simulink model "Control logic"  (R2022a)
settings: Solver=VariableStepAuto  StartTime=0.0  StopTime=10.0  RelTol=1e-3
settings Model: Creator=jbn04  LastModifiedBy=jbn04

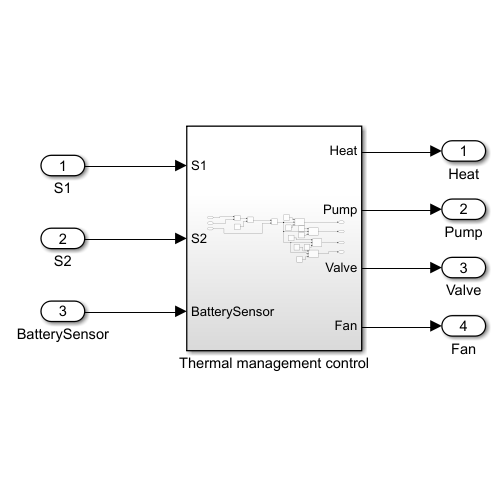
[thumbnail: Simulink's stored preview of the top-level diagram]
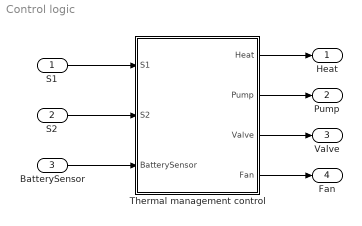
== system Control logic ==
  S1 : Inport
  S2 : Inport  Port=2
  BatterySensor : Inport  Port=3
  Thermal management control : Subsystem
  Heat : Outport
  Pump : Outport  Port=2
  Valve : Outport  Port=3
  Fan : Outport  Port=4
  wires:
  S1/1 -> Thermal management control/1(S1)
  S2/1 -> Thermal management control/2(S2)
  BatterySensor/1 -> Thermal management control/3(BatterySensor)
  Thermal management control/1(Heat) -> Heat/1
  Thermal management control/2(Pump) -> Pump/1
  Thermal management control/3(Valve) -> Valve/1
  Thermal management control/4(Fan) -> Fan/1

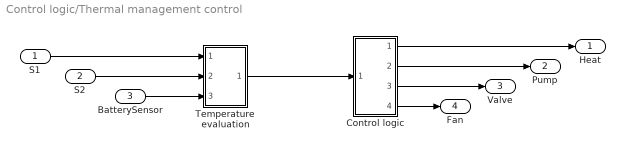
== system Control logic/Thermal management control ==
  S1 : Inport
  S2 : Inport  Port=2
  BatterySensor : Inport  Port=3
  Control logic : Subsystem
  Temperature evaluation : Subsystem
  Heat : Outport
  Pump : Outport  Port=2
  Valve : Outport  Port=3
  Fan : Outport  Port=4
  wires:
  S1/1 -> Temperature evaluation/1(In1)
  S2/1 -> Temperature evaluation/2(In2)
  BatterySensor/1 -> Temperature evaluation/3(In3)
  Temperature evaluation/1(Out1) -> Control logic/1(In1)
  Control logic/1(Out1) -> Heat/1
  Control logic/2(Out2) -> Pump/1
  Control logic/3(Out3) -> Valve/1
  Control logic/4(Out4) -> Fan/1

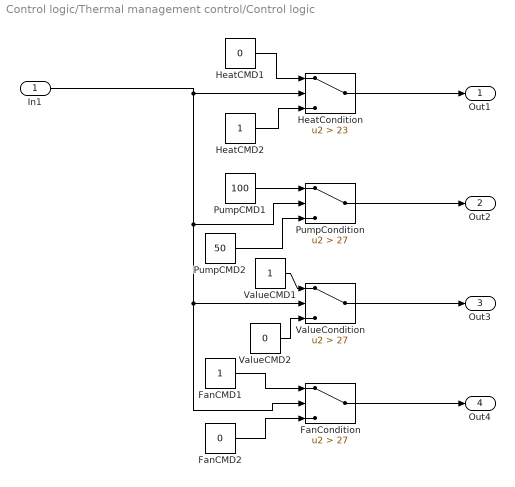
== system Control logic/Thermal management control/Control logic ==
  In1 : Inport
  FanCMD1 : Constant
  FanCMD2 : Constant  Value=0
  FanCondition : Switch  Criteria=u2 > Threshold  Threshold=27  SaturateOnIntegerOverflow=off  InputSameDT=off
  HeatCMD1 : Constant  Value=0
  HeatCMD2 : Constant
  HeatCondition : Switch  Criteria=u2 > Threshold  Threshold=23  SaturateOnIntegerOverflow=off  InputSameDT=off
  PumpCMD1 : Constant  Value=100
  PumpCMD2 : Constant  Value=50
  PumpCondition : Switch  Criteria=u2 > Threshold  Threshold=27  SaturateOnIntegerOverflow=off  InputSameDT=off
  ValueCMD1 : Constant
  ValueCMD2 : Constant  Value=0
  ValueCondition : Switch  Criteria=u2 > Threshold  Threshold=27  SaturateOnIntegerOverflow=off  InputSameDT=off
  Out1 : Outport
  Out2 : Outport  Port=2
  Out3 : Outport  Port=3
  Out4 : Outport  Port=4
  wires:
  In1/1 -> HeatCondition/2, PumpCondition/2, FanCondition/2, ValueCondition/2
  PumpCMD1/1 -> PumpCondition/1
  ValueCMD1/1 -> ValueCondition/1
  ValueCMD2/1 -> ValueCondition/3
  FanCMD1/1 -> FanCondition/1
  PumpCMD2/1 -> PumpCondition/3
  HeatCondition/1 -> Out1/1
  FanCMD2/1 -> FanCondition/3
  HeatCMD2/1 -> HeatCondition/3
  HeatCMD1/1 -> HeatCondition/1
  FanCondition/1 -> Out4/1
  PumpCondition/1 -> Out2/1
  ValueCondition/1 -> Out3/1

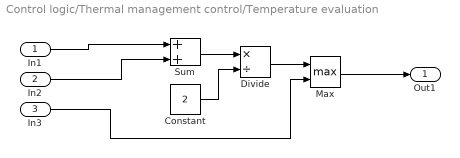
== system Control logic/Thermal management control/Temperature evaluation ==
  In1 : Inport
  In2 : Inport  Port=2
  In3 : Inport  Port=3
  Constant : Constant  Value=2
  Divide : Product  Inputs=*/
  Max : MinMax  Function=max  Inputs=2
  Sum : Sum
  Out1 : Outport
  wires:
  Divide/1 -> Max/1
  Max/1 -> Out1/1
  Sum/1 -> Divide/1
  In2/1 -> Sum/2
  In1/1 -> Sum/1
  Constant/1 -> Divide/2
  In3/1 -> Max/2
